simulink subsystem "EncoderVelocidad"  (R2023b)
settings: Solver=VariableStepAuto  StartTime=0.0  StopTime=10.0  RelTol=1e-3
libraries: arduinosensorlib x2, simulink x1
settings Model: Creator=Andrés  LastModifiedBy=Andrés

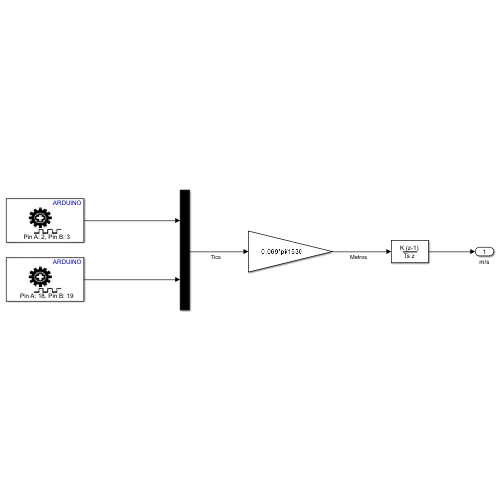
[thumbnail: Simulink's stored preview of the top-level diagram]
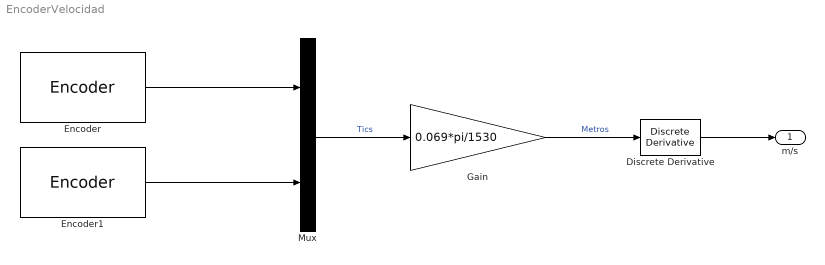
== system EncoderVelocidad ==
  Discrete Derivative : simulink/Discrete/Discrete Derivative  gainval=1.0  ICPrevScaledInput=0.0  OutMin=[]  OutMax=[]  OutDataType=fixdt(1, 16)  OutScaling=2^-10  DoSatur=off
  Encoder : arduinosensorlib/Encoder  InputA=2  InputB=3  Mode=No reset  SampleTime=-1
  Encoder1 : arduinosensorlib/Encoder  InputA=18  InputB=19  Mode=No reset  SampleTime=-1
  Gain : Gain  Gain=0.069*pi/1530  OutDataTypeStr=double
  Mux : Mux  Inputs=2
  m/s : Outport
  wires:
  Encoder/1 -> Mux/1
  Encoder1/1 -> Mux/2
  Mux/1 -> Gain/1  "Tics"
  Gain/1 -> Discrete Derivative/1  "Metros"
  Discrete Derivative/1 -> m/s/1
